simulink model "test_actuator_sensor_block"  (R2016a)
settings: Solver=VariableStepAuto  StartTime=0.0  StopTime=.15  RelTol=1e-5
settings Model: Creator=manuel  LastModifiedBy=manuel

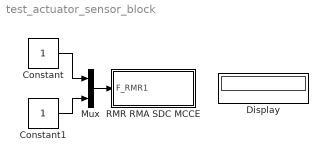
== system test_actuator_sensor_block ==
  Constant : Constant
  Constant1 : Constant
  Display : Display
  Mux : Mux  Inputs=2
  RMR RMA SDC MCCE : Subsystem
  wires:
  Mux/1 -> RMR RMA SDC MCCE/1(F_RMR1)
  Constant/1 -> Mux/1
  Constant1/1 -> Mux/2
  ? -> Display/1

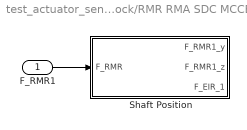
== system test_actuator_sensor_block/RMR RMA SDC MCCE ==
  F_RMR1 : Inport
  Shaft Position : MATLAB Function  TreatAsAtomicUnit=on
  wires:
  F_RMR1/1 -> Shaft Position/1(F_RMR)

== matlab function test_actuator_sensor_block/RMR RMA SDC MCCE/Shaft Position ==
  data: F_RMR input; F_RMR1_y output; F_RMR1_z output; F_EIR_1 output
function [F_RMR1_y, F_RMR1_z, F_EIR_1]  = fcn(F_RMR)
%#codegen
%%SDC1_dx, RMA1_dx, RMR1_dy, RMR1_dz, SDC1_dy, SDC1_dz, MCCE1_dz, SDC2_dx, RMA2_dx, RMR2_dy, RMR2_dz, SDC2_dy, SDC2_dz, MCCE2_dz

F_RMR1_y = F_RMR(1);
F_RMR1_z = F_RMR(2);
F_EIR_1 = 0; 

F_r = sqrt(F_RMR(1)^2 + F_RMR(2)^2)

if (F_RMR(1) ~= 0)
    theta = rad2deg(atan(F_RMR(2)/F_RMR(1)));
else
    theta = 0;
end

alpha = 360/6;

if(abs(theta) < alpha/2)
    F_EIR_1 = F_r(cos(theta) - sin(theta))/tan(alpha); 
end
